simulink model "control_light"  (R2016b)
settings: Solver=FixedStepAuto  StartTime=0.0  StopTime=10.0  RelTol=1e-3  EnableMultiTasking=on
undefined symbols (not defined in the file): Light
libraries: legoev3lib x4
settings Model: ExtModeTrigDuration=2  Creator=Nexel  LastModifiedBy=Nexel
settings SolverCC: PositivePriorityOrder=on
settings OptimizationCC: MaxStackSize=64
settings DebuggingCC: ParameterTunabilityLossMsg=error
settings HardwareCC: ProdBitPerPointer=32  ProdBitPerSizeT=32  ProdBitPerPtrDiffT=32  ProdLargestAtomicInteger=Long  ProdWordSize=32  ProdHWDeviceType=ARM Compatible->ARM 9
settings RTWCC: SystemTargetFile=ert.tlc  HardwareBoard=LEGO MINDSTORMS EV3  TLCOptions="-aInlineSetEventsForThisBaseRateFcn=TLC_FALSE -aSuppressMultiTaskScheduler=TLC_FALSE  -aRateBasedStepFcn=0"  TemplateMakefile=ert_default_tmf  Description=Embedded Coder  GenerateReport=on  Toolchain=Sourcery G++ Lite v2009q3  IncludeHyperlinkInReport=on  LaunchReport=on  GenerateTraceInfo=on  GenerateTraceReport=on  GenerateTraceReportSl=on  GenerateTraceReportSf=on  GenerateTraceReportEml=on
settings CodeAppCC: ForceParamTrailComments=on  IgnoreCustomStorageClasses=off  OperatorAnnotations=on  SimulinkDataObjDesc=on  SFDataObjDesc=on  MATLABFcnDesc=on  InsertBlockDesc=on  MATLABSourceComments=on
settings ERTTargetCC: SupportContinuousTime=on  SupportVariableSizeSignals=on

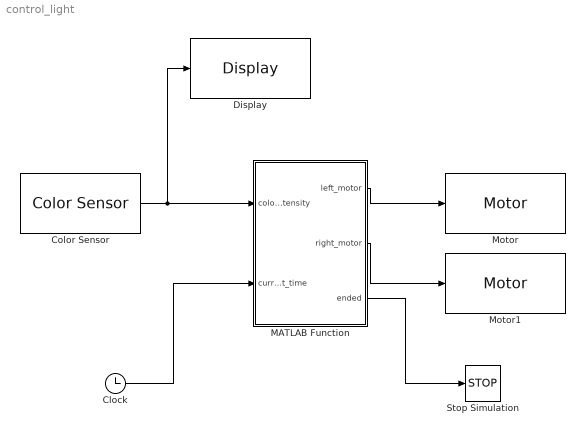
== system control_light ==
  Clock : Clock
  Color Sensor : legoev3lib/Color Sensor  portNumber=1  mode=Reflected light intensity  sampleTime=0.1
  Display : legoev3lib/Display  slcdStr=Light:  slcdLine=2  slcdFormat=Decimal
  MATLAB Function : MATLAB Function  TreatAsAtomicUnit=on
  Motor : legoev3lib/Motor  sportNumber=B  sstopAction=Brake
  Motor1 : legoev3lib/Motor  sportNumber=C  sstopAction=Brake
  Stop Simulation : Stop
  wires:
  Clock/1 -> MATLAB Function/2(current_time)
  Color Sensor/1 -> Display/1, MATLAB Function/1(color_intensity)
  MATLAB Function/1(left_motor) -> Motor/1
  MATLAB Function/2(right_motor) -> Motor1/1
  MATLAB Function/3(ended) -> Stop Simulation/1

== matlab function control_light/MATLAB Function ==
  data: color_intensity input; left_motor output; current_time input; right_motor output; ended output
function [left_motor, right_motor, ended] = control(color_intensity, current_time)
    persistent times;
    persistent intensities;
    persistent counter;
    if isempty(times)
        counter = 1;
        times = zeros(2000,1);
        intensities = zeros(2000,1);
    end
    if(current_time < 5000)
        times(counter) = current_time; intensities(counter) = color_intensity;
        ended = 0;
        R = 55;
        U = 5;
        P = 20;
        if color_intensity < R - U 
            left_motor = -P;
            right_motor = P;
        elseif color_intensity > R + U
            left_motor = P;
            right_motor = -P;
        else
            left_motor = P;
            right_motor = P;
        end
        pause(10);
    elseif(current_time == 5000)
        left_motor = 0;
        right_motor = 0;
        file = fopen('output.txt','w');
        for i = 1:length(times)
            fprintf(file, '%f \t %f', times(i,1), intensities(i,1));
        end
        fclose(file);
        ended = 1;
    else
        left_motor = 0;
        right_motor = 0;
        ended = 0;
   end
    
end
